simulink model "self_balancing_robot_sim_old"  (R2022b)
settings: Solver=VariableStepAuto  StartTime=0.0  StopTime=20  RelTol=1e-3
libraries: cstblocks x3
settings Model: Creator=antor  LastModifiedBy=antor

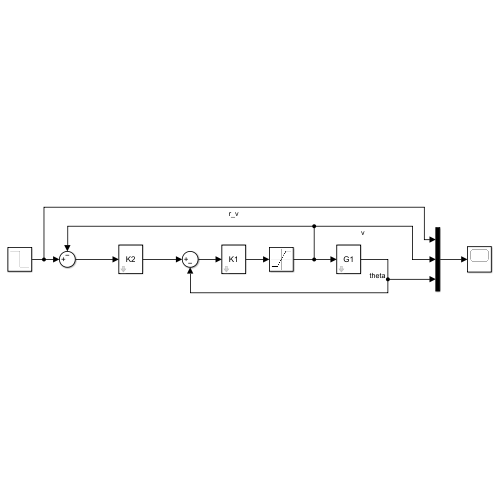
[thumbnail: Simulink's stored preview of the top-level diagram]
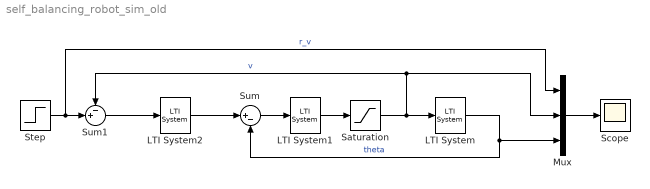
== system self_balancing_robot_sim_old ==
  LTI System : cstblocks/LTI System  sys=G1  IC=[]
  LTI System1 : cstblocks/LTI System  sys=K1  IC=[]
  LTI System2 : cstblocks/LTI System  sys=K2  IC=[]
  Mux : Mux  Inputs=3
  Saturation : Saturate  UpperLimit=20  LowerLimit=-20
  Scope : Scope
  Step : Step  Time=10  Before=10  After=0  SampleTime=0
  Sum : Sum  Inputs=|+-
  Sum1 : Sum  Inputs=-+|
  wires:
  LTI System1/1 -> Saturation/1
  Sum1/1 -> LTI System2/1
  Sum/1 -> LTI System1/1
  LTI System2/1 -> Sum/1
  LTI System/1 -> Mux/3, Sum/2  "theta"
  Step/1 -> Mux/1, Sum1/2  "r_v"
  Mux/1 -> Scope/1
  Saturation/1 -> Sum1/1, Mux/2, LTI System/1  "v"
